simulink model "stm32f4_advance_pwm_demo"  (Simulink 7.3)
settings: Solver=FixedStepDiscrete  SolverMode=SingleTasking  StartTime=0.0  StopTime=10.0  RelTol=1e-3
PreLoadFcn:
  | waijung.modelPreload; % Required for working with Waijung Blockset. Do not remove.
undefined symbols (not defined in the file): HSEOSC, Link, LQFP176, ST, STM32F417IG
libraries: stm32f4_pwm_lib x2, stm32f4_device_config_lib x1
CloseFcn:
  | waijung.modelClose; % Required for working with Waijung Blockset. Do not remove.
settings Model: Creator=Krisada  LastModifiedBy=Krisada
settings OptimizationCC: OptimizeModelRefInitCode=on  LifeSpan=1
settings HardwareCC: ProdEndianess=LittleEndian  ProdHWDeviceType=ARM Compatible->Cortex - M4  TargetEndianess=LittleEndian  TargetHWDeviceType=ARM Compatible->Cortex - M4
settings RTWCC: SystemTargetFile=stm32f4.tlc  GenerateMakefile=off  TemplateMakefile=ert_default_tmf  Description=STM32F4 Target  ProcessScript=stm32f4_make_rtw_hook
settings CodeAppCC: IgnoreCustomStorageClasses=off
settings STFCustomTargetCC: ModelReferenceCompliant=off  CombineOutputUpdateFcns=on  ERTCustomFileBanners=on  SupportContinuousTime=off  SupportNonInlinedSFcns=off  SystemTargetFile=stm32f4.tlc
settings ERTTargetCC: MultiwordLength=2048  ModelReferenceCompliant=off  ParMdlRefBuildCompliant=off  CompOptLevelCompliant=off  ERTFirstTimeCompliant=off  ModelStepFunctionPrototypeControlCompliant=off  CPPClassGenCompliant=off  InlinedParameterPlacement=NonHierarchical  ERTSrcFileBannerTemplate=stm32f4_code_template.cgt  ERTHdrFileBannerTemplate=stm32f4_code_template.cgt  ERTDataSrcFileTemplate=stm32f4_code_template.cgt  ERTDataHdrFileTemplate=stm32f4_code_template.cgt  ERTCustomFileTemplate=stm32f4_file_process.tlc

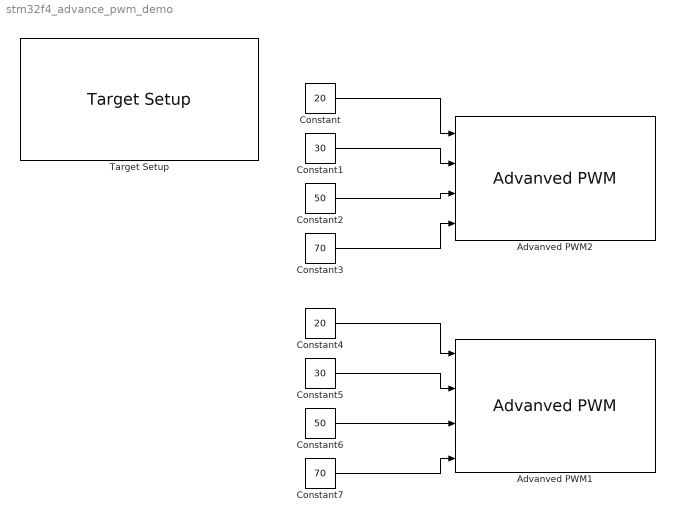
== system stm32f4_advance_pwm_demo ==
  Advanved PWM1 : stm32f4_pwm_lib/Advanved PWM  timer=TIM8  setting=Basic  period=1e-5  countermode=TIM_CounterMode_Up  use_deadtime=on  deadtime=1e-006  locklevel=TIM_LOCKLevel_OFF  breakinput=Disable  automaticoutputenable=OFF  opstate=Output and Output_N state Enable  op1=Polarity HIGH and SET when idle  op1n=Polarity HIGH and SET when idle  op2=Polarity HIGH and SET when idle  op2n=Polarity HIGH and SET when idle  op3=Polarity HIGH and SET when idle  op3n=Polarity HIGH and SET when idle  op4=Polarity HIGH and SET when idle  sampletime=-1  pwm_period=1679  pwm_presc=0  pwm_deadtime=148  blockid=AdvanvedPWM1
  Advanved PWM2 : stm32f4_pwm_lib/Advanved PWM  timer=TIM1  setting=Basic  period=1e-5  countermode=TIM_CounterMode_Up  use_deadtime=on  deadtime=1e-006  locklevel=TIM_LOCKLevel_OFF  breakinput=Disable  automaticoutputenable=OFF  opstate=Output and Output_N state Enable  op1=Polarity HIGH and SET when idle  op1n=Polarity HIGH and SET when idle  op2=Polarity HIGH and SET when idle  op2n=Polarity HIGH and SET when idle  op3=Polarity HIGH and SET when idle  op3n=Polarity HIGH and SET when idle  op4=Polarity HIGH and SET when idle  sampletime=-1  pwm_period=1679  pwm_presc=0  pwm_deadtime=148  blockid=AdvanvedPWM2
  Constant : Constant  Value=20  OutDataType=fixdt(1, 16)  OutScaling=2^0
  Constant1 : Constant  Value=30  OutDataType=fixdt(1, 16)  OutScaling=2^0
  Constant2 : Constant  Value=50  OutDataType=fixdt(1, 16)  OutScaling=2^0
  Constant3 : Constant  Value=70  OutDataType=fixdt(1, 16)  OutScaling=2^0
  Constant4 : Constant  Value=20  OutDataType=fixdt(1, 16)  OutScaling=2^0
  Constant5 : Constant  Value=30  OutDataType=fixdt(1, 16)  OutScaling=2^0
  Constant6 : Constant  Value=50  OutDataType=fixdt(1, 16)  OutScaling=2^0
  Constant7 : Constant  Value=70  OutDataType=fixdt(1, 16)  OutScaling=2^0
  Target Setup : stm32f4_device_config_lib/Target Setup  Priority=100  compiler=GNU ARM  previous_compiler=GNU ARM  mcu=STM32F417IG (LQFP176)  mcustr=STM32F417IG  clockconfig=HSEOSC-8MHz  system_stm32f4xx_c_path=F:\trunk\targets\stm32f4_target\stm32f4\utils\system_stm32f4xx_default\STM32F40_41xxx\hseosc8mhz  showmemoryconfiguration=off  stacksize=0x400  heapsize=0x200  enableautocompiledownload=on  fullchiperase=off  programmerinterface=ST-Link  editctrlstr=on  compilercontrolstr=$(patsubst %, -I%, .) -mcpu=cortex-m4 -mthumb -mthumb-interwork -mfloat-abi=hard -mfpu=fpv4-sp-d16 -ffast-math -Wall -Wextra -Ofast  assemblercontrolstr=$(patsubst %, -I%, .) -mcpu=cortex-m4 -mthumb -mthumb-interwork -mfloat-abi=hard -mfpu=fpv4-sp-d16 -ffast-math -Wall -Wextra -Ofast -Wa,-amhls=$(<:.s=.lst) -D__STACK_SIZE=$(STACK_SIZE) -D__HEAP_SIZE=$(HEAP_SIZE)  linkercontrolstr=-T$(LD_SCRIPT) -g -Wl,-Map=$(MAP),--cref,--no-warn-mismatch -mcpu=cortex-m4 -mthumb -mthumb-interwork -mfloat-abi=hard -mfpu=fpv4-sp-d16  runafterdownload=on  execprofile=None  profileruart=3  profilerbaud=115200  profilertxpin=D8  profilerinitstr=0.01,168000000,1680000,115200,0  manualsetsampletime=off  sampletime=0.01  blockid=TargetSetup  systickreloadvalue=1680000  hseval=8000000  lastprofileruart=3  hclk=168000000  flashorigin=0x8000000  flashlength=1024k  ramorigin=0x20000000  ramlength=128k  useextram=off
  wires:
  Constant/1 -> Advanved PWM2/1
  Constant1/1 -> Advanved PWM2/2
  Constant2/1 -> Advanved PWM2/3
  Constant3/1 -> Advanved PWM2/4
  Constant4/1 -> Advanved PWM1/1
  Constant5/1 -> Advanved PWM1/2
  Constant6/1 -> Advanved PWM1/3
  Constant7/1 -> Advanved PWM1/4
